simulink model "controlledrectifiers"  (R2020a)
settings: Solver=VariableStepAuto  StartTime=0.0  StopTime=0.08  RelTol=1e-3
libraries: powerlib x12, dspswit3 x1
settings Model: Creator=LAP TECHNOLOGY  LastModifiedBy=LAP TECHNOLOGY

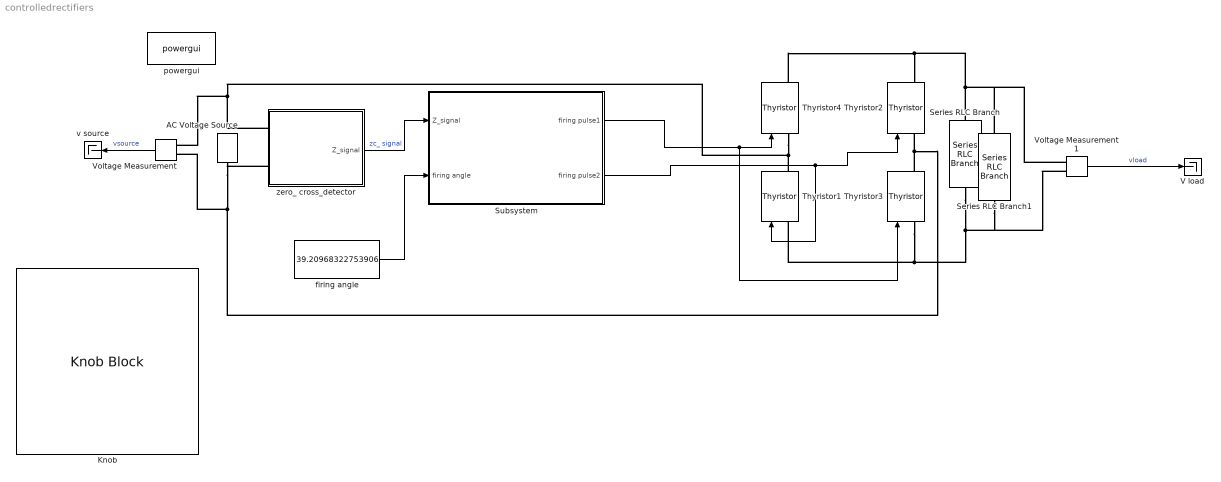
== system controlledrectifiers ==
  AC Voltage Source : powerlib/Electrical Sources/AC Voltage Source  Amplitude=sqrt(2)*220  Phase=0  Frequency=50  SampleTime=0  Measurements=None  BusType=swing  Pref=10e3  Qref=0  Qmin=-inf  Qmax=+inf
  Knob : KnobBlock  ScaleMax=180
  Series RLC Branch : powerlib/Elements/Series RLC Branch  LConnTagsString=__new0  RConnTagsString=__new0  BranchType=R  Resistance=50  Inductance=1e-3  SetiL0=off  InitialCurrent=0  Capacitance=1e-6  Setx0=off  InitialVoltage=0  Measurements=None
  Series RLC Branch1 : powerlib/Elements/Series RLC Branch  LConnTagsString=__new0  RConnTagsString=__new0  BranchType=C  Resistance=50  Inductance=1e-3  SetiL0=off  InitialCurrent=0  Capacitance=20  Setx0=off  InitialVoltage=0  Measurements=None
  Subsystem : Subsystem
  Thyristor{1..4} (4 alike) : powerlib/Power Electronics/Thyristor  Ron=0.001  Lon=0  Vf=0.8  IC=0  Rs=500  Cs=250e-9  Measurements=on
  V load : Terminator
  Voltage Measurement : powerlib/Measurements/Voltage Measurement  PhasorSimulation=off  OutputType=Complex  PSBequivalent=0
  Voltage Measurement1 : powerlib/Measurements/Voltage Measurement  PhasorSimulation=off  OutputType=Complex  PSBequivalent=0
  firing angle : Constant  Value=39.20968322753906
  powergui : powerlib/powergui  Priority=1  SimulationMode=Continuous  SampleTime=50e-6  frequency=60  Iterations=50  frequencyindice=50  Pbase=100e6  ErrMax=1e-4  UnitsV=kV  UnitsW=MW  buscounter=0  FunctionMessages=off  echomessages=off  EnableUseOfTLC=off  CurrentSourceSwitches=off  DisableSnubberDevices=off  DisableRonSwitches=off  DisableVfSwitches=off  DisplayEquations=off  AutomaticDiscreteSolvers=off  SolverType=Tustin/Backward Euler (TBE)  Interpol=off  ExternalGateDelay=off  methode=off  Ts=100  x0status=blocks  SPID=on  SwTol=0  HookPort=off  NonlinearTolerance=1e-4  nMaxIteration=100  ContinueOnMaxIteration=off  RestoreLinks=warning  ResistiveCurrentMeasurement=off  Frange=[0:2:500]  Ylog=off  Xlog=on  ShowGrid=off  save=off  variable=ZData  structure=0  ZoomFFT=off  StartTime=0.0  cycles=1  DisplayStyle=1  fundamental=60  FreqAxis=off  MaxFrequency=1000  frequencyindicesteady=1  RmsSteady=1  display=off
  v source : Terminator
  zero_ cross_detector : Subsystem
  wires:
  Subsystem/2(firing pulse2) -> Thyristor2/1, Thyristor1/1
  Subsystem/1(firing pulse1) -> Thyristor4/1, Thyristor3/1
  Voltage Measurement1/1 -> V load/1  "vload"
  Voltage Measurement/1 -> v source/1  "vsource"
  zero_ cross_detector/1("Z_signal ") -> Subsystem/1("Z_signal ")  "zc_ signal"
  firing angle/1 -> Subsystem/2("firing angle ")
  connections:
  Voltage Measurement1/LConn1 -- Series RLC Branch1/LConn1 -- Series RLC Branch/LConn1 -- Thyristor4/RConn1 -- Thyristor2/RConn1
  Thyristor1/RConn1 -- Thyristor4/LConn1 -- zero_ cross_detector/LConn1 -- Voltage Measurement/LConn2
  Thyristor3/LConn1 -- Series RLC Branch1/RConn1 -- Voltage Measurement1/LConn2 -- Series RLC Branch/RConn1 -- Thyristor1/LConn1
  Thyristor3/RConn1 -- AC Voltage Source/LConn1 -- zero_ cross_detector/LConn2 -- Voltage Measurement/LConn1 -- Thyristor2/LConn1

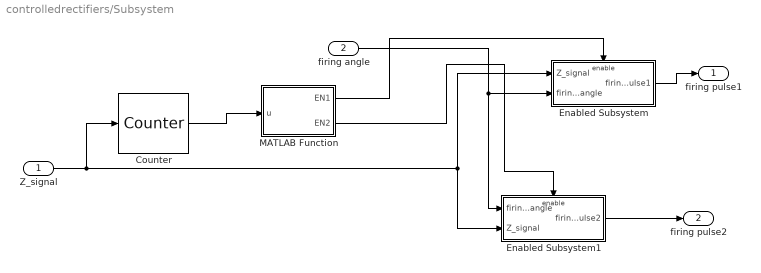
== system controlledrectifiers/Subsystem ==
  "Z_signal " : Inport
  "firing angle " : Inport  Port=2
  Counter : dspswit3/Counter  Direction=Up  CountEvent=Rising edge  CounterSize=User defined  MaxCount=255  InitialCount=0  Output=Count  HitValue=32  ResetInput=off  SamplesPerFrame=1  Ts=1  CntDtype=double  HitDtype=Logical
  Enabled Subsystem : Subsystem  TreatAsAtomicUnit=on
  Enabled Subsystem1 : Subsystem  TreatAsAtomicUnit=on
  MATLAB Function : MATLAB Function  TreatAsAtomicUnit=on
  firing pulse1 : Outport
  firing pulse2 : Outport  Port=2
  wires:
  "Z_signal "/1 -> Enabled Subsystem1/2("Z_signal "), Enabled Subsystem/1("Z_signal "), Counter/1
  Counter/1 -> MATLAB Function/1(u)
  MATLAB Function/1(EN1) -> Enabled Subsystem/Enable
  MATLAB Function/2(EN2) -> Enabled Subsystem1/Enable
  "firing angle "/1 -> Enabled Subsystem/2("firing angle "), Enabled Subsystem1/1("firing angle ")
  Enabled Subsystem/1(firing pulse1) -> firing pulse1/1
  Enabled Subsystem1/1(firing pulse2) -> firing pulse2/1

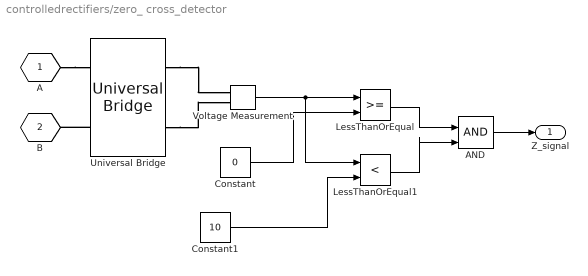
== system controlledrectifiers/zero_ cross_detector ==
  AND : Logic  IconShape=distinctive  AllPortsSameDT=off  OutDataTypeStr=boolean
  Constant : Constant  Value=0
  Constant1 : Constant  Value=10
  LessThanOrEqual : RelationalOperator  OutDataTypeStr=boolean  RndMeth=Simplest
  LessThanOrEqual1 : RelationalOperator  Operator=<  OutDataTypeStr=boolean  RndMeth=Simplest
  Universal Bridge : powerlib/Power Electronics/Universal Bridge  Arms=2  SnubberResistance=1e5  SnubberCapacitance=inf  Device=Diodes  Ron=1e-3  Lon=0  ForwardVoltages="[  0  0  ]"  ForwardVoltage=0  GTOparameters=[ 10e-6 , 20e-6 ]  IGBTparameters=[ 1e-6 , 2e-6 ]  Measurements=None  Measurements_2=None  converterType=Rectifier
  Voltage Measurement : powerlib/Measurements/Voltage Measurement  PhasorSimulation=off  OutputType=Complex  PSBequivalent=0
  A : PMIOPort  Tag=PMCPort  Side=Left
  B : PMIOPort  Tag=PMCPort  Port=2  Side=Left
  "Z_signal " : Outport
  wires:
  Voltage Measurement/1 -> LessThanOrEqual1/1, LessThanOrEqual/1
  Constant/1 -> LessThanOrEqual/2
  Constant1/1 -> LessThanOrEqual1/2
  LessThanOrEqual/1 -> AND/1
  LessThanOrEqual1/1 -> AND/2
  AND/1 -> "Z_signal "/1
  connections:
  A/RConn1 -- Universal Bridge/LConn1
  Universal Bridge/LConn2 -- B/RConn1
  Universal Bridge/RConn1 -- Voltage Measurement/LConn1
  Universal Bridge/RConn2 -- Voltage Measurement/LConn2

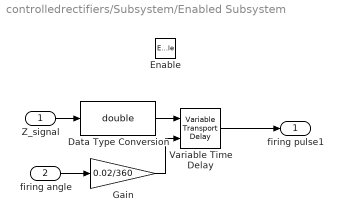
== system controlledrectifiers/Subsystem/Enabled Subsystem ==
  "Z_signal " : Inport
  "firing angle " : Inport  Port=2
  Enable : EnablePort
  Data Type Conversion : DataTypeConversion  OutDataTypeStr=double
  Gain : Gain  Gain=0.02/360
  Variable Time Delay : VariableTransportDelay  MaximumDelay=10
  firing pulse1 : Outport
  wires:
  Gain/1 -> Variable Time Delay/2
  Variable Time Delay/1 -> firing pulse1/1
  "firing angle "/1 -> Gain/1
  Data Type Conversion/1 -> Variable Time Delay/1
  "Z_signal "/1 -> Data Type Conversion/1

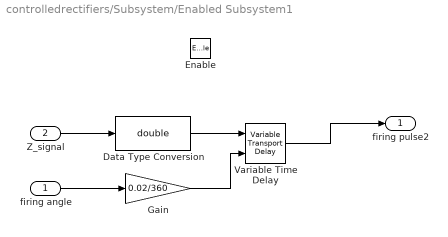
== system controlledrectifiers/Subsystem/Enabled Subsystem1 ==
  "firing angle " : Inport
  "Z_signal " : Inport  Port=2
  Enable : EnablePort
  Data Type Conversion : DataTypeConversion  OutDataTypeStr=double
  Gain : Gain  Gain=0.02/360
  Variable Time Delay : VariableTransportDelay  MaximumDelay=10
  firing pulse2 : Outport
  wires:
  Gain/1 -> Variable Time Delay/2
  Data Type Conversion/1 -> Variable Time Delay/1
  "firing angle "/1 -> Gain/1
  "Z_signal "/1 -> Data Type Conversion/1
  Variable Time Delay/1 -> firing pulse2/1

== matlab function controlledrectifiers/Subsystem/MATLAB Function ==
  data: u input; EN1 output; EN2 output
function [EN1,EN2] = fcn(u)
EN1=0;
EN2=0;

if mod(u,2)==0
    EN1=1;
    EN2=0;
    
end 
if mod(u,2)==1
    EN1=0;
    EN2=1;
end
